simulink model "ETC_model"  (R2017b)
settings: Solver=VariableStepAuto  StartTime=0.0  StopTime=10.0  RelTol=1e-3
settings Model: Creator=carca  LastModifiedBy=carca

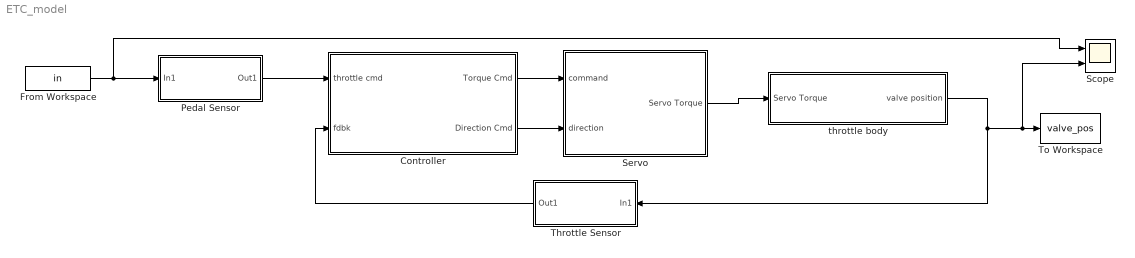
== system ETC_model ==
  Controller : Subsystem  Variant=on
  From Workspace : FromWorkspace  VariableName=in  SampleTime=0
  Pedal Sensor : Subsystem  Variant=on  OverrideUsingVariant=Variant
  Scope : Scope  NumInputPorts=2
  Servo : Subsystem  Variant=on  OverrideUsingVariant=Variant
  Throttle Sensor : Subsystem  Variant=on  OverrideUsingVariant=Variant
  To Workspace : ToWorkspace  VariableName=valve_pos  SampleTime=-1
  throttle body : Subsystem  Variant=on
  wires:
  Servo/1("Servo Torque ") -> throttle body/1(Servo Torque)
  throttle body/1(valve position) -> Scope/2, To Workspace/1, Throttle Sensor/1(In1)
  Controller/1(Torque Cmd) -> Servo/1(command)
  From Workspace/1 -> Scope/1, Pedal Sensor/1(In1)
  Controller/2(Direction Cmd) -> Servo/2(direction)
  Pedal Sensor/1(Out1) -> Controller/1(throttle cmd)
  Throttle Sensor/1(Out1) -> Controller/2(fdbk)

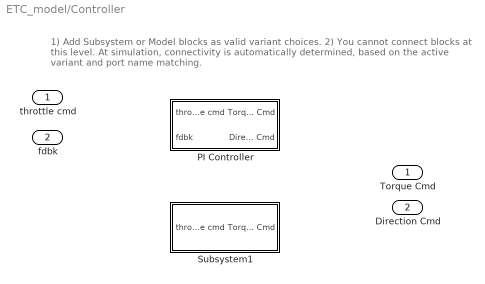
== system ETC_model/Controller ==
  note: 1) Add Subsystem or Model blocks as valid variant choices.
      | 2) You cannot connect blocks at this level. At simulation, connectivity is automatically
      | determined, based on the active variant and port name matching.
  throttle cmd : Inport
  fdbk : Inport  Port=2
  PI Controller : Subsystem  VariantControl=CTRL == 0
  Subsystem1 : Subsystem  VariantControl=CTRL == 1
  Torque Cmd : Outport
  Direction Cmd : Outport  Port=2

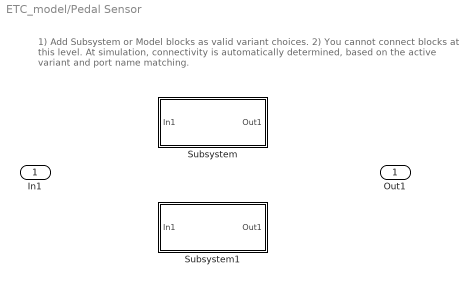
== system ETC_model/Pedal Sensor ==
  note: 1) Add Subsystem or Model blocks as valid variant choices.
      | 2) You cannot connect blocks at this level. At simulation, connectivity is automatically
      | determined, based on the active variant and port name matching.
  In1 : Inport
  Subsystem : Subsystem  VariantControl=Variant
  Subsystem1 : Subsystem  VariantControl=Variant1
  Out1 : Outport

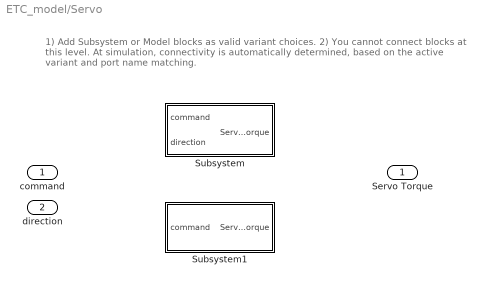
== system ETC_model/Servo ==
  note: 1) Add Subsystem or Model blocks as valid variant choices.
      | 2) You cannot connect blocks at this level. At simulation, connectivity is automatically
      | determined, based on the active variant and port name matching.
  command : Inport
  direction : Inport  Port=2
  Subsystem : Subsystem  VariantControl=Variant
  Subsystem1 : Subsystem  VariantControl=Variant1
  "Servo Torque " : Outport

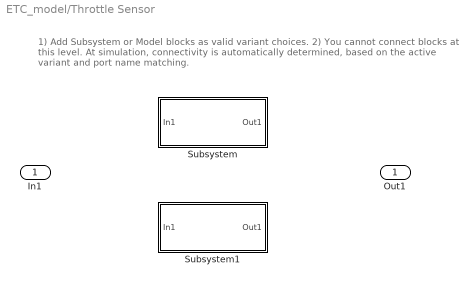
== system ETC_model/Throttle Sensor ==
  note: 1) Add Subsystem or Model blocks as valid variant choices.
      | 2) You cannot connect blocks at this level. At simulation, connectivity is automatically
      | determined, based on the active variant and port name matching.
  In1 : Inport
  Subsystem : Subsystem  VariantControl=Variant
  Subsystem1 : Subsystem  VariantControl=Variant1
  Out1 : Outport

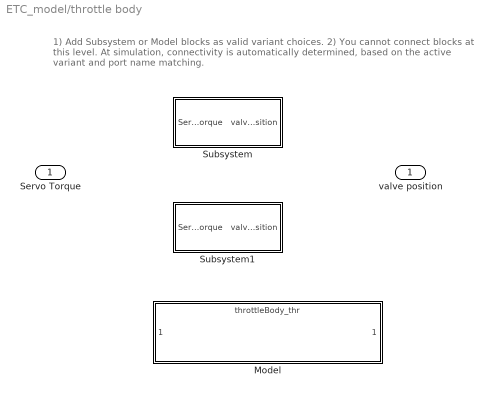
== system ETC_model/throttle body ==
  note: 1) Add Subsystem or Model blocks as valid variant choices.
      | 2) You cannot connect blocks at this level. At simulation, connectivity is automatically
      | determined, based on the active variant and port name matching.
  Servo Torque : Inport
  Model : ModelReference  ModelNameDialog=throttleBody_thr.slx  SimulationMode=Normal  VariantControl=THR == 2  ModelReferenceVersion=1.11
  Subsystem : Subsystem  VariantControl=THR == 0
  Subsystem1 : Subsystem  VariantControl=THR == 1
  valve position : Outport

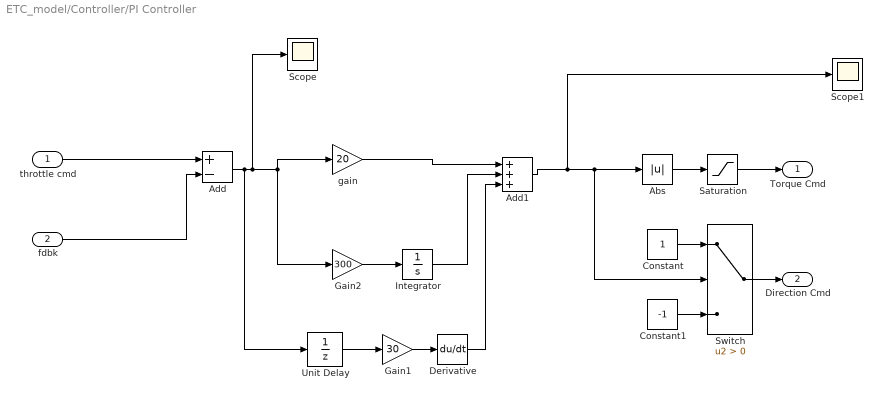
== system ETC_model/Controller/PI Controller ==
  throttle cmd : Inport
  fdbk : Inport  Port=2
  Abs : Abs
  Add : Sum  Inputs=+-
  Add1 : Sum  Inputs=+++
  Constant : Constant
  Constant1 : Constant  Value=-1
  Derivative : Derivative
  Gain1 : Gain  Gain=30
  Gain2 : Gain  Gain=300
  Integrator : Integrator
  Saturation : Saturate  UpperLimit=1  LowerLimit=0
  Scope : Scope
  Scope1 : Scope
  Switch : Switch  Criteria=u2 > Threshold
  Unit Delay : UnitDelay  SampleTime=-1
  gain : Gain  Gain=20
  Torque Cmd : Outport
  Direction Cmd : Outport  Port=2
  wires:
  Gain2/1 -> Integrator/1
  gain/1 -> Add1/1
  Integrator/1 -> Add1/2
  Add1/1 -> Scope1/1, Switch/2, Abs/1
  Abs/1 -> Saturation/1
  Constant/1 -> Switch/1
  Constant1/1 -> Switch/3
  Switch/1 -> Direction Cmd/1
  throttle cmd/1 -> Add/1
  Add/1 -> Unit Delay/1, Scope/1, Gain2/1, gain/1
  fdbk/1 -> Add/2
  Unit Delay/1 -> Gain1/1
  Gain1/1 -> Derivative/1
  Derivative/1 -> Add1/3
  Saturation/1 -> Torque Cmd/1

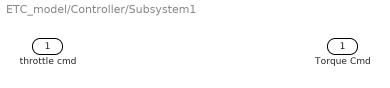
== system ETC_model/Controller/Subsystem1 ==
  throttle cmd : Inport
  Torque Cmd : Outport

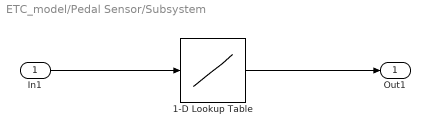
== system ETC_model/Pedal Sensor/Subsystem ==
  In1 : Inport
  1-D Lookup Table : Lookup_n-D  NumberOfTableDimensions=1  BreakpointsForDimension1=[0,90]  Table=[0,1]  InternalRulePriority=Speed  RndMeth=Simplest  InputSameDT=on
  Out1 : Outport
  wires:
  In1/1 -> 1-D Lookup Table/1
  1-D Lookup Table/1 -> Out1/1

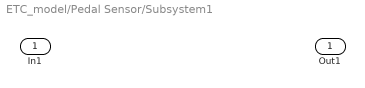
== system ETC_model/Pedal Sensor/Subsystem1 ==
  In1 : Inport
  Out1 : Outport

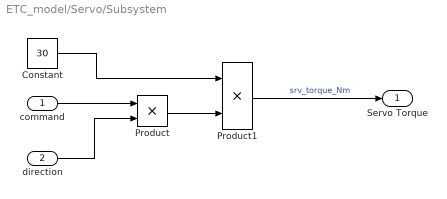
== system ETC_model/Servo/Subsystem ==
  command : Inport
  direction : Inport  Port=2
  Constant : Constant  Value=30
  Product : Product
  Product1 : Product
  "Servo Torque " : Outport
  wires:
  command/1 -> Product/1
  Product/1 -> Product1/2
  Constant/1 -> Product1/1
  Product1/1 -> "Servo Torque "/1  "srv_torque_Nm"
  direction/1 -> Product/2

== system ETC_model/Servo/Subsystem1 ==
  command : Inport
  "Servo Torque " : Outport

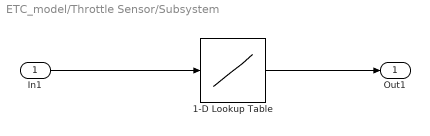
== system ETC_model/Throttle Sensor/Subsystem ==
  In1 : Inport
  1-D Lookup Table : Lookup_n-D  NumberOfTableDimensions=1  BreakpointsForDimension1=[0,90]  Table=[0,1]  InternalRulePriority=Speed  RndMeth=Simplest  InputSameDT=on
  Out1 : Outport
  wires:
  In1/1 -> 1-D Lookup Table/1
  1-D Lookup Table/1 -> Out1/1

== system ETC_model/Throttle Sensor/Subsystem1 ==
  In1 : Inport
  Out1 : Outport

== system ETC_model/throttle body/Subsystem ==
  Servo Torque : Inport
  valve position : Outport

== system ETC_model/throttle body/Subsystem1 ==
  Servo Torque : Inport
  valve position : Outport
